simulink model "linearization_scheme_HW"  (R2021a)
settings: Solver=VariableStepAuto  StartTime=0.0  StopTime=7  RelTol=1e-3
values from neighbouring files (symbols this model uses):
  a_sin = [pi/2; pi/2; 0.2; pi/2]    [HW_par.m]
  delta = 1/sqrt(2)    [HW_par.m]
  Kd = 1000*eye(4)    [HW_par.m]
  Kp = 10000*eye(4)    [HW_par.m]
  omega_sin = 0.5*[1; 1; 1; 1]    [HW_par.m]
  q_0 = [0;0;0;0]    [HW_par.m]
  q_dot_0 = [0;0;0;0]    [HW_par.m]
  w_c = 2*pi*50    (= 314.159265359)    [HW_par.m]
undefined symbols (not defined in the file or in its folder): a_filt, b_filt
settings Model: Creator=jacop_  LastModifiedBy=jacop_

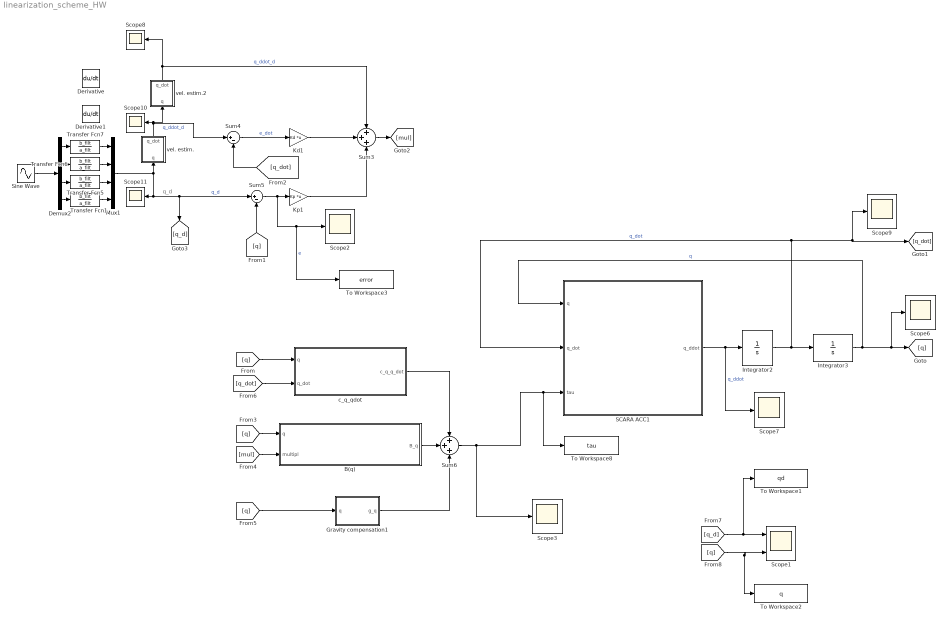
== system linearization_scheme_HW ==
  note: q_d
  B(q) : MATLAB Function  TreatAsAtomicUnit=on
  Demux2 : Demux
  Derivative : Derivative
  Derivative1 : Derivative
  Gravity compensation1 : MATLAB Function  TreatAsAtomicUnit=on
  Integrator2 : Integrator  InitialCondition=q_dot_0
  Integrator3 : Integrator  InitialCondition=q_0
  Kd1 : Gain  Gain=Kd  Multiplication=Matrix(K*u)
  Kp1 : Gain  Gain=Kp  Multiplication=Matrix(K*u)
  Mux1 : Mux
  SCARA ACC1 : MATLAB Function  TreatAsAtomicUnit=on
  Scope1 : Scope  NumInputPorts=2
  Scope{2..3,6..11} (8 alike) : Scope
  Sine Wave : Sin  Amplitude=a_sin  Frequency=omega_sin  SampleTime=0
  Sum3 : Sum  Inputs=+++
  Sum4 : Sum  Inputs=|+-
  Sum5 : Sum  Inputs=|+-
  Sum6 : Sum  Inputs=+++
  To Workspace1 : ToWorkspace  VariableName=qd  SaveFormat=Structure With Time  SampleTime=-1
  To Workspace2 : ToWorkspace  VariableName=q  SaveFormat=Structure With Time  SampleTime=-1
  To Workspace3 : ToWorkspace  VariableName=error  SaveFormat=Structure With Time  SampleTime=-1
  To Workspace8 : ToWorkspace  VariableName=tau  SaveFormat=Structure With Time  SampleTime=-1
  Transfer Fcn{1,5..7} (4 alike) : TransferFcn  Numerator=b_filt  Denominator=a_filt
  c_q_qdot : MATLAB Function  TreatAsAtomicUnit=on
  vel. estim. : Subsystem
  vel. estim.2 : Subsystem
  wires:
  Transfer Fcn1/1 -> Mux1/4
  Transfer Fcn5/1 -> Mux1/3
  SCARA ACC1/1(q_ddot) -> Integrator2/1, Scope7/1  "q_ddot"
  Transfer Fcn6/1 -> Mux1/2
  Kd1/1 -> Sum3/2
  Integrator3/1 -> [q], Scope6/1, SCARA ACC1/1(q)  "q"
  Mux1/1 -> vel. estim./1(q), [q_d], Sum5/1, Scope11/1  "q_d"
  Demux2/1 -> Transfer Fcn7/1
  Sum4/1 -> Kd1/1  "e_dot"
  Sine Wave/1 -> Demux2/1
  Demux2/3 -> Transfer Fcn5/1
  Sum5/1 -> To Workspace3/1, Scope2/1, Kp1/1  "e"
  Gravity compensation1/1(g_q) -> Sum6/3
  Demux2/2 -> Transfer Fcn6/1
  Demux2/4 -> Transfer Fcn1/1
  Kp1/1 -> Sum3/3
  Transfer Fcn7/1 -> Mux1/1
  vel. estim.2/1(q_dot) -> Scope8/1, Sum3/1  "q_ddot_d"
  Integrator2/1 -> Integrator3/1, SCARA ACC1/2(q_dot), [q_dot], Scope9/1  "q_dot"
  Sum6/1 -> Scope3/1, To Workspace8/1, SCARA ACC1/3(tau)
  [q] -> c_q_qdot/1(q)
  [q] -> Sum5/2
  c_q_qdot/1(c_q_q_dot) -> Sum6/1
  B(q)/1(B_q) -> Sum6/2
  [q_dot] -> Sum4/2
  [q] -> B(q)/1(q)
  Sum3/1 -> [mul]
  [mul] -> B(q)/2(multipl)
  [q] -> Gravity compensation1/1(q)
  [q_dot] -> c_q_qdot/2(q_dot)
  [q] -> To Workspace2/1, Scope1/2
  [q_d] -> To Workspace1/1, Scope1/1
  vel. estim./1(q_dot) -> Sum4/1, vel. estim.2/1(q), Scope10/1  "q_ddot_d"

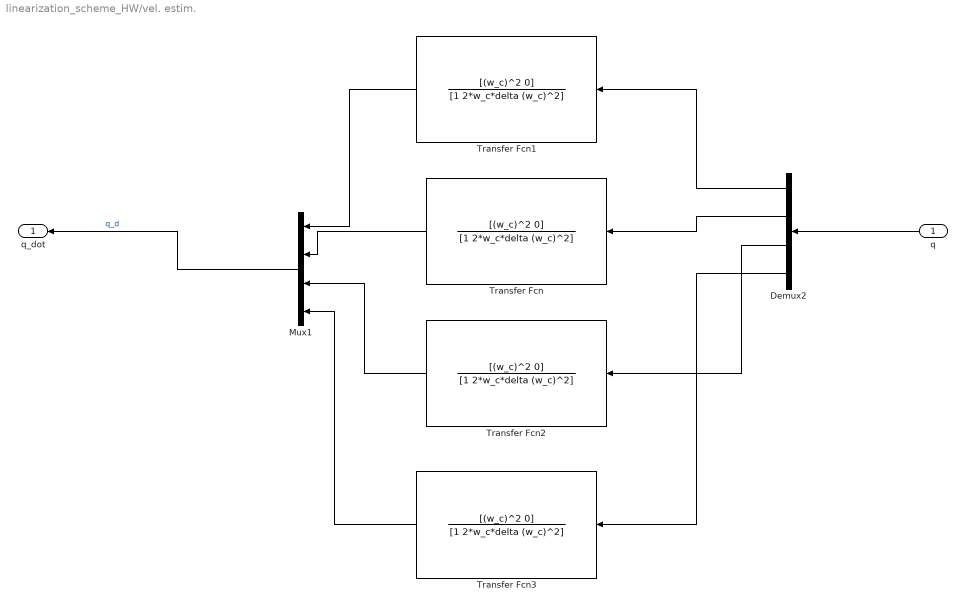
== system linearization_scheme_HW/vel. estim. ==
  q : Inport
  Demux2 : Demux
  Mux1 : Mux
  Transfer Fcn{,1..3} (4 alike) : TransferFcn  Numerator=[(w_c)^2 0]  Denominator=[1 2*w_c*delta (w_c)^2]
  q_dot : Outport
  wires:
  q/1 -> Demux2/1
  Demux2/4 -> Transfer Fcn3/1
  Demux2/3 -> Transfer Fcn2/1
  Demux2/2 -> Transfer Fcn/1
  Demux2/1 -> Transfer Fcn1/1
  Transfer Fcn/1 -> Mux1/2
  Transfer Fcn1/1 -> Mux1/1
  Transfer Fcn2/1 -> Mux1/3
  Transfer Fcn3/1 -> Mux1/4
  Mux1/1 -> q_dot/1  "q_d"

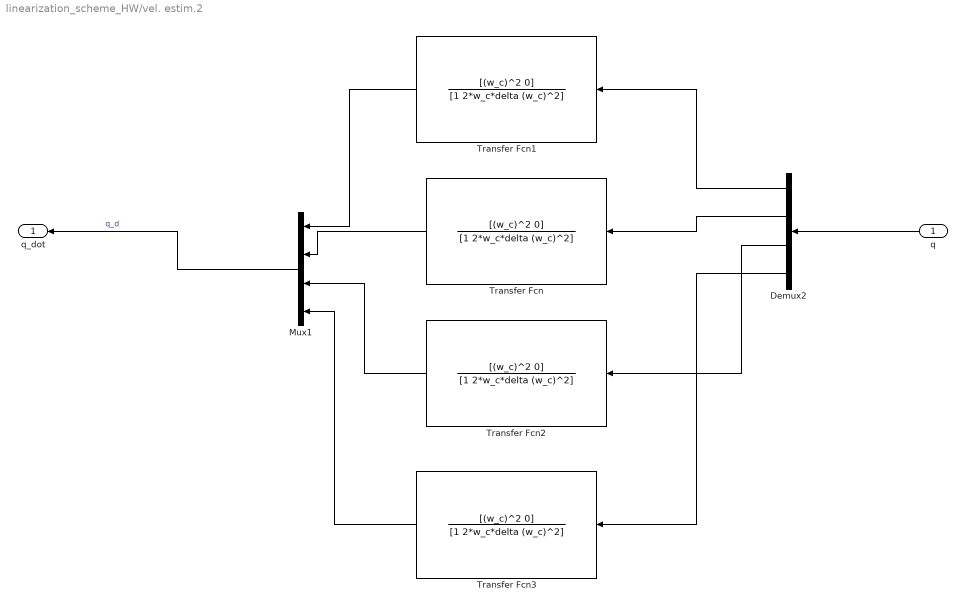
== system linearization_scheme_HW/vel. estim.2 ==
  q : Inport
  Demux2 : Demux
  Mux1 : Mux
  Transfer Fcn{,1..3} (4 alike) : TransferFcn  Numerator=[(w_c)^2 0]  Denominator=[1 2*w_c*delta (w_c)^2]
  q_dot : Outport
  wires:
  Mux1/1 -> q_dot/1  "q_d"
  Transfer Fcn3/1 -> Mux1/4
  Transfer Fcn2/1 -> Mux1/3
  Transfer Fcn1/1 -> Mux1/1
  Transfer Fcn/1 -> Mux1/2
  Demux2/1 -> Transfer Fcn1/1
  Demux2/2 -> Transfer Fcn/1
  Demux2/3 -> Transfer Fcn2/1
  Demux2/4 -> Transfer Fcn3/1
  q/1 -> Demux2/1

== matlab function linearization_scheme_HW/SCARA ACC1 ==
  data: q input; q_ddot output; q_dot input; tau input
function q_ddot = SCARA_acc(q, q_dot, tau)%#codegen
coder.extrinsic('f_B_mex'); 
coder.extrinsic('f_C_vect_mex'); 
coder.extrinsic('f_g_vect_mex');
B = eye(4);
C_vect = zeros(4,1);
F_g = zeros(4,1);
tau = reshape(tau,4,1);
q_ddot = zeros(4,1);
B = full(f_B_mex('f_B',q));
C_vect = full(f_C_vect_mex('f_C_vect', q, q_dot));
F_g = full(f_g_vect_mex('f_g_vect', q));
q_ddot = (eye(4)/B)*(-C_vect-F_g+tau);

== matlab function linearization_scheme_HW/c_q_qdot ==
  data: q input; c_q_q_dot output; q_dot input
function c_q_q_dot = c_q_qdot_term(q, q_dot)
coder.extrinsic('f_C_vect_mex'); 
C_vect = zeros(4,1);
C_vect = full(f_C_vect_mex('f_C_vect', q, q_dot));
c_q_q_dot = C_vect;

== matlab function linearization_scheme_HW/B(q) ==
  data: q input; B_q output; multipl input
function B_q = B_q_term(q, multipl)
coder.extrinsic('f_B_mex'); 
B = eye(4);
B_q = zeros(4,1);
multipl = reshape( multipl,4,1);
B = full(f_B_mex('f_B',q));
B_q = B*multipl;

== matlab function linearization_scheme_HW/Gravity compensation1 ==
  data: q input; g_q output
function g_q = g_q_term(q)
coder.extrinsic('f_g_vect_mex');
F_g = zeros(4,1);
g_q = zeros(4,1);
F_g = full(f_g_vect_mex('f_g_vect', q));
g_q = F_g;
